simulink model "simu"  (R2019b)
settings: Solver=VariableStepAuto  StartTime=0.0  StopTime=1  RelTol=1e-3
(part 1 of 2)
settings Model: Creator=deepa  LastModifiedBy=deepa

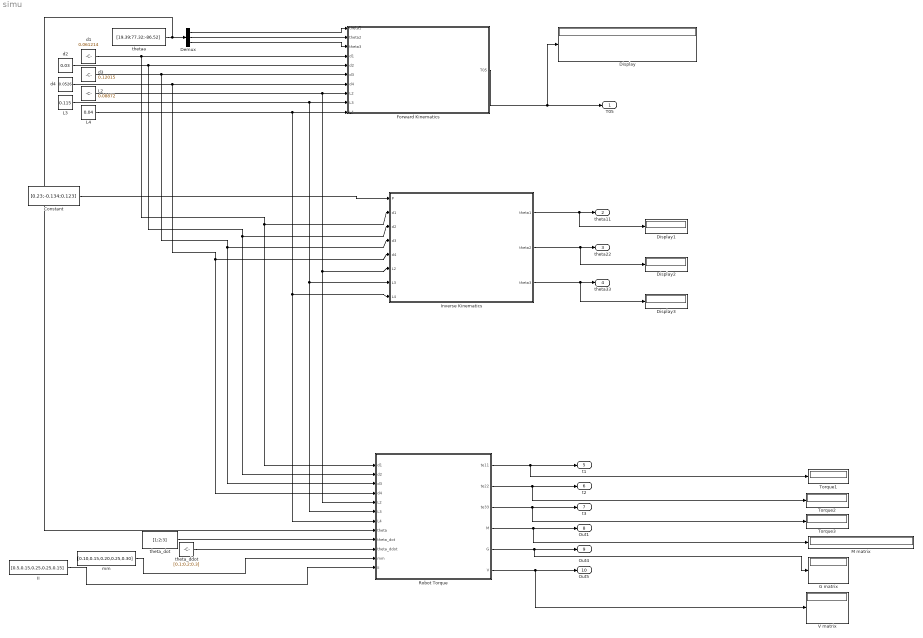
== system simu ==
  Constant : Constant  Value=[0.23;-0.134;0.123]
  Demux : Demux  Outputs=3
  Display{,1..3} (4 alike) : Display
  "Forward Kinematics " : MATLAB Function  TreatAsAtomicUnit=on
  G matrix : Display
  "II " : Constant  Value=[0.5,0.15,0.25,0.25,0.15]
  "Inverse Kinematics " : MATLAB Function  TreatAsAtomicUnit=on
  L2 : Constant  Value=0.08872
  L3 : Constant  Value=0.115
  L4 : Constant  Value=0.04
  M matrix : Display
  "Robot Torque " : MATLAB Function  TreatAsAtomicUnit=on
  Torque1 : Display
      settings: Decimation=4
  Torque2 : Display
  "Torque3 " : Display
  "V matrix " : Display
  d1 : Constant  Value=0.061214
  d2 : Constant  Value=0.03
  d3 : Constant  Value=0.12015
  d4 : Constant  Value=0.0526
  "mm " : Constant  Value=[0.10,0.15,0.20,0.25,0.30]
  "theta_ddot " : Constant  Value=[0.1;0.2;0.3]
  "theta_dot " : Constant  Value=[1;2;3]
  "thetaa " : Constant  Value=[19.39;77.32;-86.52]
  "T05 " : Outport
  theta11 : Outport  Port=2
  theta22 : Outport  Port=3
  theta33 : Outport  Port=4
  t1 : Outport  Port=5
  t2 : Outport  Port=6
  t3 : Outport  Port=7
  Out1 : Outport  Port=8
  Out4 : Outport  Port=9
  Out5 : Outport  Port=10
  wires:
  d1/1 -> "Robot Torque "/1(d1), "Inverse Kinematics "/2(d1), "Forward Kinematics "/4(d1)
  d3/1 -> "Robot Torque "/3(d3), "Inverse Kinematics "/4(d3), "Forward Kinematics "/6(d3)
  d4/1 -> "Robot Torque "/4(d4), "Inverse Kinematics "/5(d4), "Forward Kinematics "/7(d4)
  L2/1 -> "Robot Torque "/5(L2), "Inverse Kinematics "/6(L2), "Forward Kinematics "/8(L2)
  L3/1 -> "Robot Torque "/6(L3), "Inverse Kinematics "/7(L3), "Forward Kinematics "/9(L3)
  L4/1 -> "Robot Torque "/7(L4), "Inverse Kinematics "/8(L4), "Forward Kinematics "/10(L4)
  "thetaa "/1 -> "Robot Torque "/8(theta), Demux/1
  Demux/1 -> "Forward Kinematics "/1(theta1)
  Demux/2 -> "Forward Kinematics "/2(theta2)
  Demux/3 -> "Forward Kinematics "/3(theta3)
  d2/1 -> "Robot Torque "/2(d2), "Inverse Kinematics "/3(d2), "Forward Kinematics "/5(d2)
  "Inverse Kinematics "/1(theta1) -> Display1/1, theta11/1
  "Inverse Kinematics "/2(theta2) -> Display2/1, theta22/1
  "Inverse Kinematics "/3(theta3) -> Display3/1, theta33/1
  "Forward Kinematics "/1(T05) -> "T05 "/1, Display/1
  "theta_dot "/1 -> "Robot Torque "/9(theta_dot)
  "theta_ddot "/1 -> "Robot Torque "/10(theta_ddot)
  "mm "/1 -> "Robot Torque "/11(mm)
  "II "/1 -> "Robot Torque "/12(II)
  "Robot Torque "/1(te11) -> Torque1/1, t1/1
  "Robot Torque "/2(te22) -> t2/1, Torque2/1
  "Robot Torque "/3(te33) -> t3/1, "Torque3 "/1
  "Robot Torque "/4(M) -> M matrix/1, Out1/1
  "Robot Torque "/5(G) -> G matrix/1, Out4/1
  "Robot Torque "/6(V) -> Out5/1, "V matrix "/1
  Constant/1 -> "Inverse Kinematics "/1(P)

== matlab function simu/Inverse Kinematics  ==
  data: P input; theta1 output; d1 input; d2 input; d3 input; d4 input; L2 input; L3 input; L4 input; theta2 output; theta3 output
function [theta1,theta2,theta3] = inverse_kinematic(P,d1, d2, d3,d4, L2, L3, L4)
    Px = P(1);Py= P(2); Pz =P(3);
    alpha =0;
    alpha1 = asind(-Py/sqrt((Px^2 +Py^2)));
    alpha2 = acosd(Px/sqrt((Px^2+Py^2)));
    if Px>0 
       alpha = alpha1; 
    else
       alpha = alpha2;
    end
    theta1 = asind((d2+d3+d4)/sqrt((Px^2 +Py^2)))-alpha;
    K2 = Pz - d1;
    K1 = Px*cosd(theta1) + Py*sind(theta1) ;
    c3 = ((K1^2 + K2^2-(L3+L4)^2-L2^2)/(2*L2*(L3+L4)));
    s3 = sqrt(1-(c3^2));
    theta3 = -acosd(c3);
    s2 = ((K2*(L2+(L3+L4)*cosd(theta3)))-(K1*(L3+L4)*sind(theta3)))/(((L3+L4)*sind(theta3))^2+(L2+(L3+L4)*cosd(theta3))^2);
    c2 = (K1+(L3+L4)*s2*sind(theta3))/(L2+(L3+L4)*cosd(theta3));
    theta2 = atan2d(s2,c2);
end

== matlab function simu/Forward Kinematics  ==
  data: theta1 input; T05 output; theta2 input; theta3 input; d1 input; d2 input; d3 input; d4 input; L2 input; L3 input; L4 input
function T05  = forward_kinematics_simu(theta1, theta2, theta3, d1, d2, d3,d4, L2, L3, L4)
    % Define the transformation matrices using Craig's convention
    T01 = CT_JcraigDEG(0, 0, d1, theta1);
    T12 = CT_JcraigDEG(90, 0, d2, theta2);
    T23 = CT_JcraigDEG(0, L2, d3, theta3);
    T34 = CT_JcraigDEG(0, L3, d4, 0);
    T45 = CT_JcraigDEG(0, L4, 0, 0);
    % Compute the overall transformation matrix
    T05 = T01 * T12 * T23 * T34 * T45;
end
